simulink model "ver1SensorModeling"  (R2020a)
settings: Solver=FixedStepAuto  StartTime=0.0  StopTime=10.0  FixedStep=1e-4  RelTol=1e-3
settings Model: Creator=Mehmet  LastModifiedBy=Mehmet

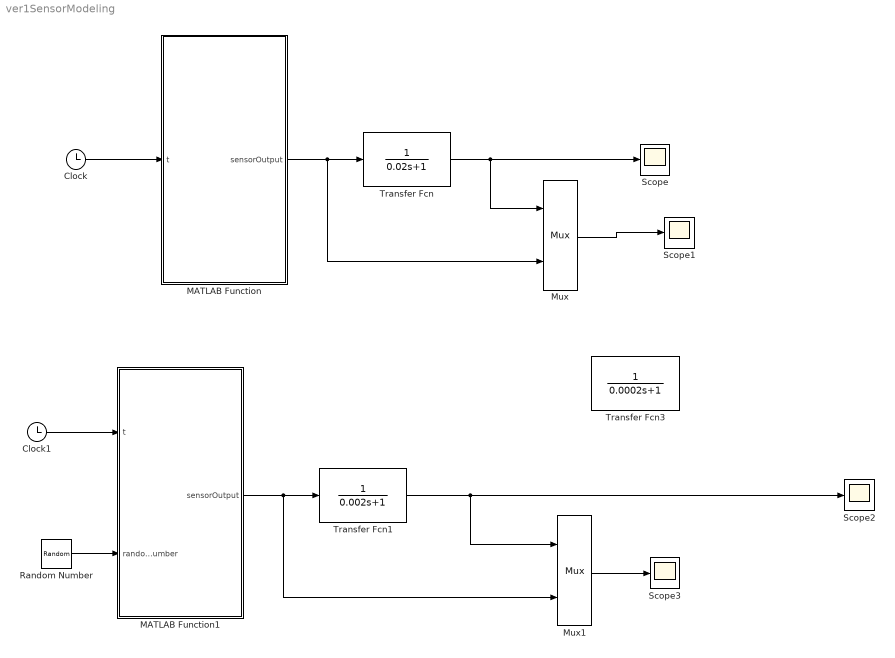
== system ver1SensorModeling ==
  Clock : Clock
  Clock1 : Clock
  MATLAB Function : MATLAB Function  TreatAsAtomicUnit=on
  MATLAB Function1 : MATLAB Function  TreatAsAtomicUnit=on
  Mux : Mux  Inputs=2
  Mux1 : Mux  Inputs=2
  Random Number : RandomNumber  Variance=0.1  SampleTime=1e-4
  Scope{,1..3} (4 alike) : Scope
  Transfer Fcn : TransferFcn  Denominator=[0.02 1]
  Transfer Fcn1 : TransferFcn  Denominator=[0.002 1]
  Transfer Fcn3 : TransferFcn  Denominator=[0.0002 1]
  wires:
  Clock/1 -> MATLAB Function/1(t)
  MATLAB Function/1(sensorOutput) -> Mux/2, Transfer Fcn/1
  Transfer Fcn/1 -> Mux/1, Scope/1
  Mux/1 -> Scope1/1
  Clock1/1 -> MATLAB Function1/1(t)
  MATLAB Function1/1(sensorOutput) -> Transfer Fcn1/1, Mux1/2
  Mux1/1 -> Scope3/1
  Transfer Fcn1/1 -> Scope2/1, Mux1/1
  Random Number/1 -> MATLAB Function1/2(randomNumber)

== matlab function ver1SensorModeling/MATLAB Function ==
  data: t input; sensorOutput output
function sensorOutput = fcn(t)

tMod = mod(t,6);

sensorOutputIn = 0;

if tMod < 2

    sensorOutputIn = 5;

end

if tMod >= 2 && tMod < 4
   
    sensorOutputIn = 3;
    
end

if tMod >= 4 && tMod < 6
   
    sensorOutputIn = 7;
    
end
    

sensorOutput = sensorOutputIn;

end

== matlab function ver1SensorModeling/MATLAB Function1 ==
  data: t input; sensorOutput output; randomNumber input
function sensorOutput = fcn(t,randomNumber)

tMod = mod(t,6);

sensorOutputIn = 0;

if tMod < 2

    sensorOutputIn = 5 + randomNumber;

end

if tMod >= 2 && tMod < 4
   
    sensorOutputIn = 3 + randomNumber;
    
end

if tMod >= 4 && tMod < 6
   
    sensorOutputIn = 7 + randomNumber;
    
end
    

sensorOutput = sensorOutputIn;

end
